simulink model "120_conduction_3ph_inverter"  (R2016b)
settings: Solver=VariableStepAuto  StartTime=0.0  StopTime=0.1  RelTol=1e-3
libraries: powerlib x21
settings Model: Creator=Yash Bansod  LastModifiedBy=Yash Bansod

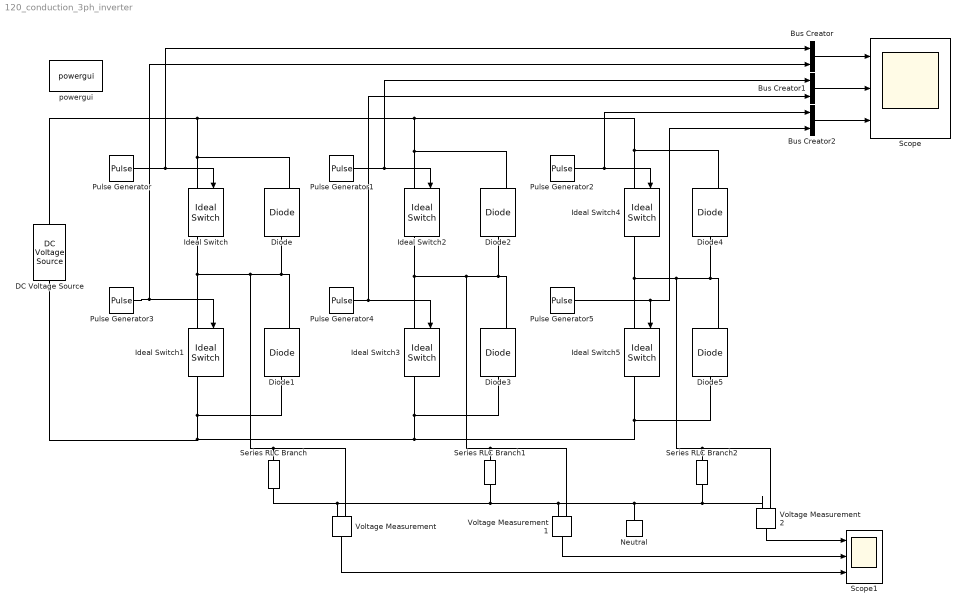
== system 120_conduction_3ph_inverter ==
  Bus Creator : BusCreator  Inputs=2
  Bus Creator1 : BusCreator  Inputs=2
  Bus Creator2 : BusCreator  Inputs=2
  DC Voltage Source : powerlib/Electrical Sources/DC Voltage Source  Amplitude=100  Measurements=Voltage
  Diode{,1..5} (6 alike) : powerlib/Power Electronics/Diode  Ron=0.001  Lon=0  Vf=0.8  IC=0  UseSnubber=off  Rs=500  Cs=250e-9  Measurements=on
  Ideal Switch{,1..5} (6 alike) : powerlib/Power Electronics/Ideal Switch  Ron=0.001  Lon=0  IC=0  Rs=1e5  Cs=inf  Measurements=on
  Neutral : powerlib/Elements/Neutral  LConnTagsString=a  NodeNumber=10
  Pulse Generator : DiscretePulseGenerator  PulseType=Time based  Period=0.02  PulseWidth=(100/3)
  Pulse Generator1 : DiscretePulseGenerator  PulseType=Time based  Period=0.02  PulseWidth=(100/3)  PhaseDelay=-(0.04/3)
  Pulse Generator2 : DiscretePulseGenerator  PulseType=Time based  Period=0.02  PulseWidth=(100/3)  PhaseDelay=-(0.02/3)
  Pulse Generator3 : DiscretePulseGenerator  PulseType=Time based  Period=0.02  PulseWidth=(100/3)  PhaseDelay=0.01
  Pulse Generator4 : DiscretePulseGenerator  PulseType=Time based  Period=0.02  PulseWidth=(100/3)  PhaseDelay=-(0.04/3)+0.01
  Pulse Generator5 : DiscretePulseGenerator  PulseType=Time based  Period=0.02  PulseWidth=(100/3)  PhaseDelay=-(0.02/3)+0.01
  Scope : Scope  NumInputPorts=3
  Scope1 : Scope  NumInputPorts=3
  Series RLC Branch : powerlib/Elements/Series RLC Branch  LConnTagsString=__new0  RConnTagsString=__new0  BranchType=R  Resistance=1  Inductance=1e-3  SetiL0=off  InitialCurrent=0  Capacitance=1e-6  Setx0=off  InitialVoltage=0  Measurements=None
  Series RLC Branch1 : powerlib/Elements/Series RLC Branch  LConnTagsString=__new0  RConnTagsString=__new0  BranchType=R  Resistance=1  Inductance=1e-3  SetiL0=off  InitialCurrent=0  Capacitance=1e-6  Setx0=off  InitialVoltage=0  Measurements=None
  Series RLC Branch2 : powerlib/Elements/Series RLC Branch  LConnTagsString=__new0  RConnTagsString=__new0  BranchType=R  Resistance=1  Inductance=1e-3  SetiL0=off  InitialCurrent=0  Capacitance=1e-6  Setx0=off  InitialVoltage=0  Measurements=None
  Voltage Measurement : powerlib/Measurements/Voltage Measurement  PhasorSimulation=off  OutputType=Complex  PSBequivalent=0
  Voltage Measurement1 : powerlib/Measurements/Voltage Measurement  PhasorSimulation=off  OutputType=Complex  PSBequivalent=0
  Voltage Measurement2 : powerlib/Measurements/Voltage Measurement  PhasorSimulation=off  OutputType=Complex  PSBequivalent=0
  powergui : powerlib/powergui  Priority=1  SimulationMode=Continuous  SolverType=Tustin/Backward Euler (TBE)  SampleTime=50e-6  frequency=60  SPID=on  DisableSnubberDevices=off  DisableRonSwitches=off  DisableVfSwitches=off  SwTol=0  DisplayEquations=off  Interpol=off  ExternalGateDelay=off  methode=off  Ts=10  FunctionMessages=off  echomessages=off  HookPort=off  EnableUseOfTLC=off  x0status=blocks  frequencyindice=0  Pbase=100e6  ErrMax=1e-4  Iterations=50  UnitsV=kV  UnitsW=MW  buscounter=0  RestoreLinks=warning  ResistiveCurrentMeasurement=off  Frange=[0:2:500]  Ylog=off  Xlog=on  ShowGrid=off  save=off  variable=ZData  structure=0  ZoomFFT=off  StartTime=0.0  cycles=1  DisplayStyle=1  fundamental=60  FreqAxis=off  MaxFrequency=1000  frequencyindicesteady=1  RmsSteady=1  display=off
  wires:
  Pulse Generator/1 -> Bus Creator/1, Ideal Switch/1
  Pulse Generator3/1 -> Bus Creator/2, Ideal Switch1/1
  Pulse Generator1/1 -> Bus Creator1/1, Ideal Switch2/1
  Pulse Generator4/1 -> Bus Creator1/2, Ideal Switch3/1
  Pulse Generator2/1 -> Bus Creator2/1, Ideal Switch4/1
  Pulse Generator5/1 -> Ideal Switch5/1, Bus Creator2/2
  Bus Creator1/1 -> Scope/2
  Bus Creator/1 -> Scope/1
  Bus Creator2/1 -> Scope/3
  Voltage Measurement2/1 -> Scope1/1
  Voltage Measurement1/1 -> Scope1/2
  Voltage Measurement/1 -> Scope1/3
  connections:
  DC Voltage Source/RConn1 -- Diode4/RConn1 -- Ideal Switch4/LConn1 -- Diode2/RConn1 -- Ideal Switch2/LConn1 -- Diode/RConn1 -- Ideal Switch/LConn1
  Ideal Switch/RConn1 -- Voltage Measurement/LConn1 -- Series RLC Branch/LConn1 -- Diode/LConn1 -- Diode1/RConn1 -- Ideal Switch1/LConn1
  Ideal Switch1/RConn1 -- Diode1/LConn1 -- Diode5/LConn1 -- Ideal Switch5/RConn1 -- Diode3/LConn1 -- Ideal Switch3/RConn1 -- DC Voltage Source/LConn1
  Ideal Switch2/RConn1 -- Voltage Measurement1/LConn1 -- Series RLC Branch1/LConn1 -- Diode2/LConn1 -- Diode3/RConn1 -- Ideal Switch3/LConn1
  Diode5/RConn1 -- Diode4/LConn1 -- Voltage Measurement2/LConn1 -- Series RLC Branch2/LConn1 -- Ideal Switch4/RConn1 -- Ideal Switch5/LConn1
  Series RLC Branch2/RConn1 -- Voltage Measurement2/LConn2 -- Neutral/LConn1 -- Voltage Measurement1/LConn2 -- Voltage Measurement/LConn2 -- Series RLC Branch/RConn1 -- Series RLC Branch1/RConn1
